simulink model "Inference_only"  (R2022a)
settings: Solver=VariableStepAuto  StartTime=0.0  StopTime=6  RelTol=1e-3
values from neighbouring files (symbols this model uses):
  num_layer = 2    [Inference_only_2x2_input.m]
undefined symbols (not defined in the file or in its folder): xc7k70tfbv676
libraries: hdlBasic x38, vmcUtilities x1
settings Model: Creator=gaozh  LastModifiedBy=gaozh

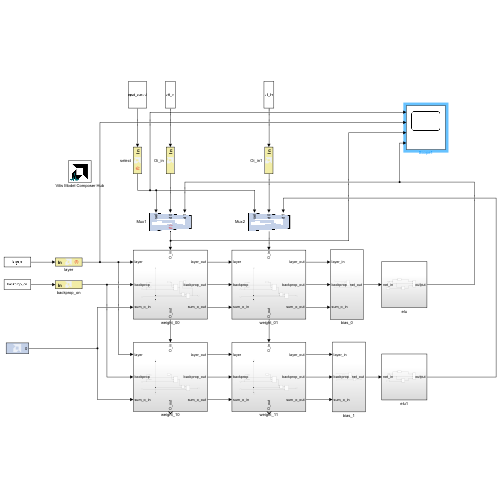
[thumbnail: Simulink's stored preview of the top-level diagram]
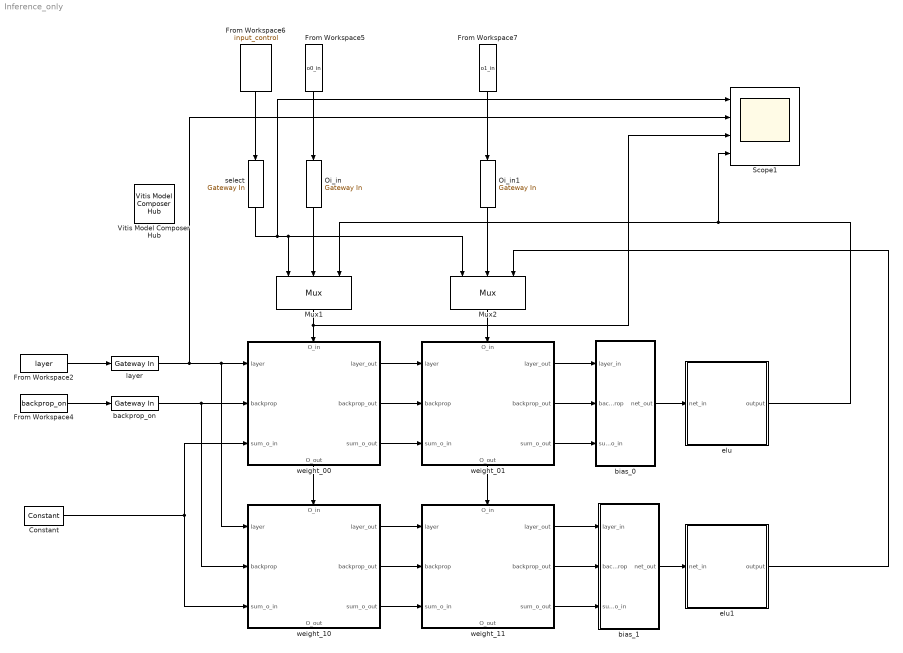
== system Inference_only ==
  Constant : hdlBasic/Constant  const=0  gui_display_data_type=Fixed-point  arith_type=Signed (2's comp)  n_bits=num_bits  bin_pt=frac_bits  preci_type=Single  exp_width=8  frac_width=24  explicit_period=off  period=1  XmcBlockStatus=1  maskContainerNames=tabcontainer1  block_type=constant  block_config=sysgen:Constant_config
  From Workspace2 : FromWorkspace  VariableName=layer
  From Workspace4 : FromWorkspace  VariableName=backprop_on
  From Workspace5 : FromWorkspace  VariableName=o0_in
  From Workspace6 : FromWorkspace  VariableName=input_control  OutputAfterFinalValue=Holding final value
  From Workspace7 : FromWorkspace  VariableName=o1_in
  Mux1 : hdlBasic/Mux  inputs=2  en=off  latency=0  precision=User Defined  arith_type="Signed  (2's comp)"  n_bits=num_bits  bin_pt=frac_bits  quantization=Truncate  overflow=Wrap  XmcBlockStatus=1  maskContainerNames=tabcontainer1  block_type=mux  block_config=sysgen:Mux_config
  Mux2 : hdlBasic/Mux  inputs=2  en=off  latency=0  precision=User Defined  arith_type="Signed  (2's comp)"  n_bits=num_bits  bin_pt=frac_bits  quantization=Truncate  overflow=Wrap  XmcBlockStatus=1  maskContainerNames=tabcontainer1  block_type=mux  block_config=sysgen:Mux_config
  Oi_in : hdlBasic/Gateway In  gui_display_data_type=Fixed-point  arith_type=Signed (2's comp)  n_bits=num_bits  bin_pt=frac_bits  preci_type=Single  exp_width=8  frac_width=24  rows=1  columns=1  quantization="Round  (unbiased: +/- Inf)"  overflow=Saturate  period=1  UseAsADC=off  ADCChannel='1'  interface=None  automatic_assignment=on  address_offset=hex2dec('00')  intf_name=''  intf_description=''  default_value=0  timing_constraint=None  locs_specified=off  LOCs={}  io_standard={}  inherit_from_input=off  hdl_port=on  XmcBlockStatus=1  maskContainerNames=group4  block_type=gatewayin  block_config=sysgen:gateway_in_config  block_width_w=590  block_height_w=620  block_width=640  block_height=850
  Oi_in1 : hdlBasic/Gateway In  gui_display_data_type=Fixed-point  arith_type=Signed (2's comp)  n_bits=num_bits  bin_pt=frac_bits  preci_type=Single  exp_width=8  frac_width=24  rows=1  columns=1  quantization="Round  (unbiased: +/- Inf)"  overflow=Saturate  period=1  UseAsADC=off  ADCChannel='1'  interface=None  automatic_assignment=on  address_offset=hex2dec('00')  intf_name=''  intf_description=''  default_value=0  timing_constraint=None  locs_specified=off  LOCs={}  io_standard={}  inherit_from_input=off  hdl_port=on  XmcBlockStatus=1  maskContainerNames=group4  block_type=gatewayin  block_config=sysgen:gateway_in_config  block_width_w=590  block_height_w=620  block_width=640  block_height=850
  Scope1 : Scope  NumInputPorts=4
  Vitis Model Composer Hub : vmcUtilities/Vitis Model Composer Hub  Tag=genX  CodeGeneration=off  TargetDirectory=./code  ExportType=AI Engines  IpVendor=xilinx.com  IpLibrary=hls  IpVersion=1.0  IpHWLanguage=Verilog  AieCompilerOptions={}  AieSimulatorOptions={}  CreateTestbench=off  TestbenchStackSize=10  RunAieSim=off  AieSimTimeout=50000  RunAieSimProfiling=off  LaunchVitisAnalyzer=off  PlotOutput=off  RunX86Sim=off  X86SimTimeout=10  GenHwImage=off  PlatformType=Not Specified  HwSystemType=Baremetal  HwValidationTarget=hw  ProjDevice=xc7k70tfbv676-1  ProjDevicePart=xc7k70tfbv676-1  SamplePeriod=-1  ClockFrequency=200  DataPathParallelism=1  xilinxfamily=kintex7  part=xc7k70t  speed=-1  package=fbv676  directory=./netlist  testbench=off  incr_netlist=off  synthesis_tool=Vivado  clock_wrapper=Clock Enables  dbl_ovrd=According to Block Masks  dcm_input_clock_period=10  sysclk_period=10  simulink_period=1  eval_field=0  IPInfoJsonString="{\"HDLSubsystem\":{\"SubsystemName\":\"PE_weightstationary\",\"IPName\":\"weight_pe\",\"IPLibrary\":\"VMC\",\"IPVendor\":\"User Company\",\"IPVersion\":\"1.0\"}}"  LogFileName=''  NThreads=4
  backprop_on : hdlBasic/Gateway In  gui_display_data_type=Boolean  arith_type=Boolean  n_bits=num_bits  bin_pt=0  preci_type=Single  exp_width=8  frac_width=24  rows=1  columns=1  quantization="Round  (unbiased: +/- Inf)"  overflow=Saturate  period=1  UseAsADC=off  ADCChannel='1'  interface=None  automatic_assignment=on  address_offset=hex2dec('00')  intf_name=''  intf_description=''  default_value=0  timing_constraint=None  locs_specified=off  LOCs={}  io_standard={}  inherit_from_input=off  hdl_port=on  XmcBlockStatus=1  maskContainerNames=group4  block_type=gatewayin  block_config=sysgen:gateway_in_config  block_width_w=590  block_height_w=620  block_width=640  block_height=850
  bias_0 : Subsystem
  bias_1 : Subsystem
  elu : Subsystem
  elu1 : Subsystem
  layer : hdlBasic/Gateway In  gui_display_data_type=Fixed-point  arith_type=Unsigned  n_bits=ceil(log2(num_layer))  bin_pt=0  preci_type=Single  exp_width=8  frac_width=24  rows=1  columns=1  quantization="Round  (unbiased: +/- Inf)"  overflow=Saturate  period=1  UseAsADC=off  ADCChannel='1'  interface=None  automatic_assignment=on  address_offset=hex2dec('00')  intf_name=''  intf_description=''  default_value=0  timing_constraint=None  locs_specified=off  LOCs={}  io_standard={}  inherit_from_input=off  hdl_port=on  XmcBlockStatus=1  maskContainerNames=group4  block_type=gatewayin  block_config=sysgen:gateway_in_config  block_width_w=590  block_height_w=620  block_width=640  block_height=850
  select : hdlBasic/Gateway In  gui_display_data_type=Fixed-point  arith_type=Unsigned  n_bits=1  bin_pt=0  preci_type=Single  exp_width=8  frac_width=24  rows=1  columns=1  quantization="Round  (unbiased: +/- Inf)"  overflow=Flag as error  period=1  UseAsADC=off  ADCChannel='1'  interface=None  automatic_assignment=on  address_offset=hex2dec('00')  intf_name=''  intf_description=''  default_value=0  timing_constraint=None  locs_specified=off  LOCs={}  io_standard={}  inherit_from_input=off  hdl_port=on  XmcBlockStatus=1  maskContainerNames=group4  block_type=gatewayin  block_config=sysgen:gateway_in_config  block_width_w=590  block_height_w=620  block_width=640  block_height=850
  weight_00 : Subsystem
      settings: PortSchema="{\"entries\":[{\"content\":{\"sides\":[{\"content\":{\"connectorIds\":[\"In1\",\"In2\",\"In3\"]},\"type\":\"ConnectorPlacement.EquallySpacedRectSide\",\"uuid\":\"632a3ded-5b94-406e-b0d8-119737680536\"},{\"content\":{\"connectorIds\":[\"Out1\",\"Out2\",\"Out3\"],\"side\":\"RIGHT\"},\"type\":\"ConnectorPlacement.EquallySpacedRectSide\",\"uuid\":\"c449027c-81bc-4843-8994-fcad26195520\"},{\"content\":{\"connectorIds\":[\"In4\"],\"side\":\"TOP\"},\"type\":\"ConnectorPlacement.EquallySpacedRectSide\",\"uuid\":\"ce3d970d-7335-434e-bfbf-286e0c492397\"},{\"content\":{\"connectorIds\":[\"Out4\"],\"side\":\"BOTTOM\"},\"type\":\"ConnectorPlacement.EquallySpacedRectSide\",\"uuid\":\"bc179919-f31d-4e0a-abc3-bb5ef913c3c8\"}]},\"type\":\"ConnectorPlacement.EquallySpacedConnector\",\"uuid\":\"cad1cfc6-1bed-4a03-a2df-30ebe0a8ed6f\"}],\"packageUris\":[\"http://schema.mathworks.com/mf0/Connector/R2020b\"],\"version\":\"1.0\"}"
  weight_01 : Subsystem
      settings: PortSchema="{\"entries\":[{\"content\":{\"sides\":[{\"content\":{\"connectorIds\":[\"In1\",\"In2\",\"In3\"]},\"type\":\"ConnectorPlacement.EquallySpacedRectSide\",\"uuid\":\"632a3ded-5b94-406e-b0d8-119737680536\"},{\"content\":{\"connectorIds\":[\"Out1\",\"Out2\",\"Out3\"],\"side\":\"RIGHT\"},\"type\":\"ConnectorPlacement.EquallySpacedRectSide\",\"uuid\":\"c449027c-81bc-4843-8994-fcad26195520\"},{\"content\":{\"connectorIds\":[\"In4\"],\"side\":\"TOP\"},\"type\":\"ConnectorPlacement.EquallySpacedRectSide\",\"uuid\":\"ce3d970d-7335-434e-bfbf-286e0c492397\"},{\"content\":{\"connectorIds\":[\"Out4\"],\"side\":\"BOTTOM\"},\"type\":\"ConnectorPlacement.EquallySpacedRectSide\",\"uuid\":\"bc179919-f31d-4e0a-abc3-bb5ef913c3c8\"}]},\"type\":\"ConnectorPlacement.EquallySpacedConnector\",\"uuid\":\"cad1cfc6-1bed-4a03-a2df-30ebe0a8ed6f\"}],\"packageUris\":[\"http://schema.mathworks.com/mf0/Connector/R2020b\"],\"version\":\"1.0\"}"
  weight_10 : Subsystem
      settings: PortSchema="{\"entries\":[{\"content\":{\"sides\":[{\"content\":{\"connectorIds\":[\"In1\",\"In2\",\"In3\"]},\"type\":\"ConnectorPlacement.EquallySpacedRectSide\",\"uuid\":\"632a3ded-5b94-406e-b0d8-119737680536\"},{\"content\":{\"connectorIds\":[\"Out1\",\"Out2\",\"Out3\"],\"side\":\"RIGHT\"},\"type\":\"ConnectorPlacement.EquallySpacedRectSide\",\"uuid\":\"c449027c-81bc-4843-8994-fcad26195520\"},{\"content\":{\"connectorIds\":[\"In4\"],\"side\":\"TOP\"},\"type\":\"ConnectorPlacement.EquallySpacedRectSide\",\"uuid\":\"ce3d970d-7335-434e-bfbf-286e0c492397\"},{\"content\":{\"connectorIds\":[\"Out4\"],\"side\":\"BOTTOM\"},\"type\":\"ConnectorPlacement.EquallySpacedRectSide\",\"uuid\":\"bc179919-f31d-4e0a-abc3-bb5ef913c3c8\"}]},\"type\":\"ConnectorPlacement.EquallySpacedConnector\",\"uuid\":\"cad1cfc6-1bed-4a03-a2df-30ebe0a8ed6f\"}],\"packageUris\":[\"http://schema.mathworks.com/mf0/Connector/R2020b\"],\"version\":\"1.0\"}"
  weight_11 : Subsystem
      settings: PortSchema="{\"entries\":[{\"content\":{\"sides\":[{\"content\":{\"connectorIds\":[\"In1\",\"In2\",\"In3\"]},\"type\":\"ConnectorPlacement.EquallySpacedRectSide\",\"uuid\":\"632a3ded-5b94-406e-b0d8-119737680536\"},{\"content\":{\"connectorIds\":[\"Out1\",\"Out2\",\"Out3\"],\"side\":\"RIGHT\"},\"type\":\"ConnectorPlacement.EquallySpacedRectSide\",\"uuid\":\"c449027c-81bc-4843-8994-fcad26195520\"},{\"content\":{\"connectorIds\":[\"In4\"],\"side\":\"TOP\"},\"type\":\"ConnectorPlacement.EquallySpacedRectSide\",\"uuid\":\"ce3d970d-7335-434e-bfbf-286e0c492397\"},{\"content\":{\"connectorIds\":[\"Out4\"],\"side\":\"BOTTOM\"},\"type\":\"ConnectorPlacement.EquallySpacedRectSide\",\"uuid\":\"bc179919-f31d-4e0a-abc3-bb5ef913c3c8\"}]},\"type\":\"ConnectorPlacement.EquallySpacedConnector\",\"uuid\":\"cad1cfc6-1bed-4a03-a2df-30ebe0a8ed6f\"}],\"packageUris\":[\"http://schema.mathworks.com/mf0/Connector/R2020b\"],\"version\":\"1.0\"}"
  wires:
  From Workspace4/1 -> backprop_on/1
  From Workspace5/1 -> Oi_in/1
  backprop_on/1 -> weight_10/2(backprop), weight_00/2(backprop)
  layer/1 -> weight_10/1(layer), weight_00/1(layer), Scope1/2
  From Workspace7/1 -> Oi_in1/1
  From Workspace2/1 -> layer/1
  Mux2/1 -> weight_01/4(O_in)
  From Workspace6/1 -> select/1
  select/1 -> Scope1/1, Mux2/1, Mux1/1
  Mux1/1 -> weight_00/4(O_in), Scope1/3
  Oi_in/1 -> Mux1/2
  Oi_in1/1 -> Mux2/2
  weight_10/2(backprop_out) -> weight_11/2(backprop)
  weight_00/2(backprop_out) -> weight_01/2(backprop)
  weight_00/3(sum_o_out) -> weight_01/3(sum_o_in)
  weight_00/1(layer_out) -> weight_01/1(layer)
  weight_10/1(layer_out) -> weight_11/1(layer)
  weight_10/3(sum_o_out) -> weight_11/3(sum_o_in)
  weight_01/4(O_out) -> weight_11/4(O_in)
  weight_00/4(O_out) -> weight_10/4(O_in)
  weight_01/1(layer_out) -> bias_0/1(layer_in)
  weight_01/2(backprop_out) -> bias_0/2(backprop)
  weight_01/3(sum_o_out) -> bias_0/3(sum_o_in)
  weight_11/1(layer_out) -> bias_1/1(layer_in)
  weight_11/3(sum_o_out) -> bias_1/3(sum_o_in)
  weight_11/2(backprop_out) -> bias_1/2(backprop)
  bias_1/1(net_out) -> elu1/1(net_in)
  elu/1(output) -> Scope1/4, Mux1/3
  elu1/1(output) -> Mux2/3
  Constant/1 -> weight_10/3(sum_o_in), weight_00/3(sum_o_in)
  bias_0/1(net_out) -> elu/1(net_in)

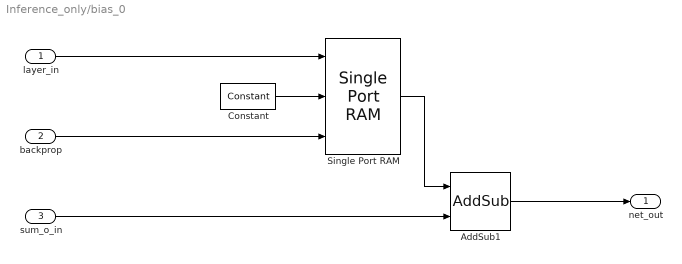
== system Inference_only/bias_0 ==
  layer_in : Inport
  backprop : Inport  Port=2
  sum_o_in : Inport  Port=3
  AddSub1 : hdlBasic/AddSub  mode=Addition  use_carryin=off  use_carryout=off  en=off  latency=0  precision=User Defined  arith_type="Signed  (2's comp)"  n_bits=num_bits  bin_pt=frac_bits  quantization=Truncate  overflow=Saturate  use_behavioral_HDL=off  hw_selection=Fabric  pipelined=off  XmcBlockStatus=1  maskContainerNames=tabcontainer1  block_type=addsub  block_config=sysgen:Addsub_config
  Constant : hdlBasic/Constant  const=0  gui_display_data_type=Fixed-point  arith_type=Signed (2's comp)  n_bits=num_bits  bin_pt=frac_bits  preci_type=Single  exp_width=8  frac_width=24  explicit_period=off  period=1  XmcBlockStatus=1  maskContainerNames=tabcontainer1  block_type=constant  block_config=sysgen:Constant_config
  Single Port RAM : hdlBasic/Single Port RAM  depth=num_layer  initVector=b1  distributed_mem=Block RAM  write_mode=Read After Write  rst=off  init_reg=0  en=off  optimize_latency=off  latency=1  optimize=Area  dbl_ovrd=off  simulation_type=fast_sim  XmcBlockStatus=1  maskContainerNames=tabcontainer1  block_type=spram  block_config=sysgen:SPRAM_config
  net_out : Outport
  wires:
  layer_in/1 -> Single Port RAM/1
  backprop/1 -> Single Port RAM/3
  sum_o_in/1 -> AddSub1/2
  Single Port RAM/1 -> AddSub1/1
  AddSub1/1 -> net_out/1
  Constant/1 -> Single Port RAM/2

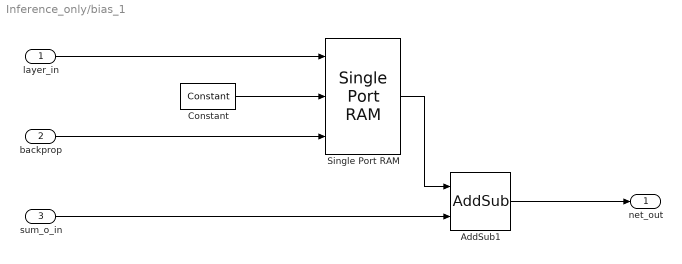
== system Inference_only/bias_1 ==
  layer_in : Inport
  backprop : Inport  Port=2
  sum_o_in : Inport  Port=3
  AddSub1 : hdlBasic/AddSub  mode=Addition  use_carryin=off  use_carryout=off  en=off  latency=0  precision=User Defined  arith_type="Signed  (2's comp)"  n_bits=num_bits  bin_pt=frac_bits  quantization=Truncate  overflow=Saturate  use_behavioral_HDL=off  hw_selection=Fabric  pipelined=off  XmcBlockStatus=1  maskContainerNames=tabcontainer1  block_type=addsub  block_config=sysgen:Addsub_config
  Constant : hdlBasic/Constant  const=0  gui_display_data_type=Fixed-point  arith_type=Signed (2's comp)  n_bits=num_bits  bin_pt=frac_bits  preci_type=Single  exp_width=8  frac_width=24  explicit_period=off  period=1  XmcBlockStatus=1  maskContainerNames=tabcontainer1  block_type=constant  block_config=sysgen:Constant_config
  Single Port RAM : hdlBasic/Single Port RAM  depth=num_layer  initVector=b2  distributed_mem=Block RAM  write_mode=Read After Write  rst=off  init_reg=0  en=off  optimize_latency=off  latency=1  optimize=Area  dbl_ovrd=off  simulation_type=fast_sim  XmcBlockStatus=1  maskContainerNames=tabcontainer1  block_type=spram  block_config=sysgen:SPRAM_config
  net_out : Outport
  wires:
  layer_in/1 -> Single Port RAM/1
  backprop/1 -> Single Port RAM/3
  sum_o_in/1 -> AddSub1/2
  Single Port RAM/1 -> AddSub1/1
  AddSub1/1 -> net_out/1
  Constant/1 -> Single Port RAM/2

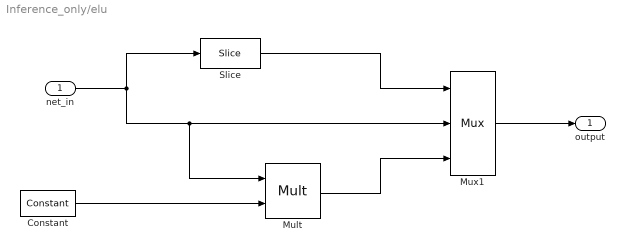
== system Inference_only/elu ==
  net_in : Inport
  Constant : hdlBasic/Constant  const=0.03  gui_display_data_type=Fixed-point  arith_type=Signed (2's comp)  n_bits=num_bits  bin_pt=frac_bits  preci_type=Single  exp_width=8  frac_width=24  explicit_period=off  period=1  XmcBlockStatus=1  maskContainerNames=tabcontainer1  block_type=constant  block_config=sysgen:Constant_config
  Mult : hdlBasic/Mult  precision=User Defined  arith_type="Signed  (2's comp)"  n_bits=num_bits  bin_pt=3  quantization=Truncate  overflow=Wrap  en=off  latency=0  use_behavioral_HDL=off  opt=Speed  use_embedded=on  optimum_pipeline=off  pipeline=on  use_rpm=on  placement_style=Triangular  XmcBlockStatus=1  maskContainerNames=group1  block_type=mult  block_config=sysgen:Mult_config  block_width=598  block_height=876
  Mux1 : hdlBasic/Mux  inputs=2  en=off  latency=1  precision=User Defined  arith_type="Signed  (2's comp)"  n_bits=num_bits  bin_pt=3  quantization=Truncate  overflow=Wrap  XmcBlockStatus=1  maskContainerNames=tabcontainer1  block_type=mux  block_config=sysgen:Mux_config
  Slice : hdlBasic/Slice  nbits=1  boolean_output=on  mode=Upper Bit Location + Width  bit1=0  base1=MSB of Input  bit0=0  base0=LSB of Input  XmcBlockStatus=1  maskContainerNames=group1  block_type=slice  block_config=sysgen:Slice_config
  output : Outport
  wires:
  Mult/1 -> Mux1/3
  Constant/1 -> Mult/2
  Slice/1 -> Mux1/1
  net_in/1 -> Slice/1, Mux1/2, Mult/1
  Mux1/1 -> output/1

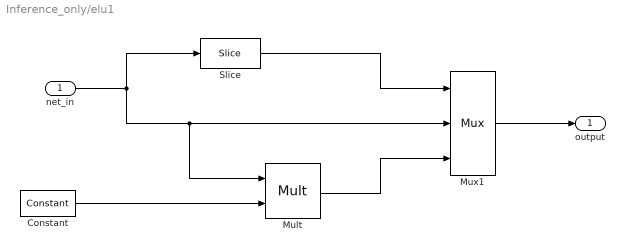
== system Inference_only/elu1 ==
  net_in : Inport
  Constant : hdlBasic/Constant  const=0.03  gui_display_data_type=Fixed-point  arith_type=Signed (2's comp)  n_bits=num_bits  bin_pt=frac_bits  preci_type=Single  exp_width=8  frac_width=24  explicit_period=off  period=1  XmcBlockStatus=1  maskContainerNames=tabcontainer1  block_type=constant  block_config=sysgen:Constant_config
  Mult : hdlBasic/Mult  precision=User Defined  arith_type="Signed  (2's comp)"  n_bits=num_bits  bin_pt=3  quantization=Truncate  overflow=Wrap  en=off  latency=0  use_behavioral_HDL=off  opt=Speed  use_embedded=on  optimum_pipeline=off  pipeline=on  use_rpm=on  placement_style=Triangular  XmcBlockStatus=1  maskContainerNames=group1  block_type=mult  block_config=sysgen:Mult_config  block_width=598  block_height=876
  Mux1 : hdlBasic/Mux  inputs=2  en=off  latency=1  precision=User Defined  arith_type="Signed  (2's comp)"  n_bits=num_bits  bin_pt=3  quantization=Truncate  overflow=Wrap  XmcBlockStatus=1  maskContainerNames=tabcontainer1  block_type=mux  block_config=sysgen:Mux_config
  Slice : hdlBasic/Slice  nbits=1  boolean_output=on  mode=Upper Bit Location + Width  bit1=0  base1=MSB of Input  bit0=0  base0=LSB of Input  XmcBlockStatus=1  maskContainerNames=group1  block_type=slice  block_config=sysgen:Slice_config
  output : Outport
  wires:
  Mult/1 -> Mux1/3
  Constant/1 -> Mult/2
  Slice/1 -> Mux1/1
  net_in/1 -> Slice/1, Mux1/2, Mult/1
  Mux1/1 -> output/1

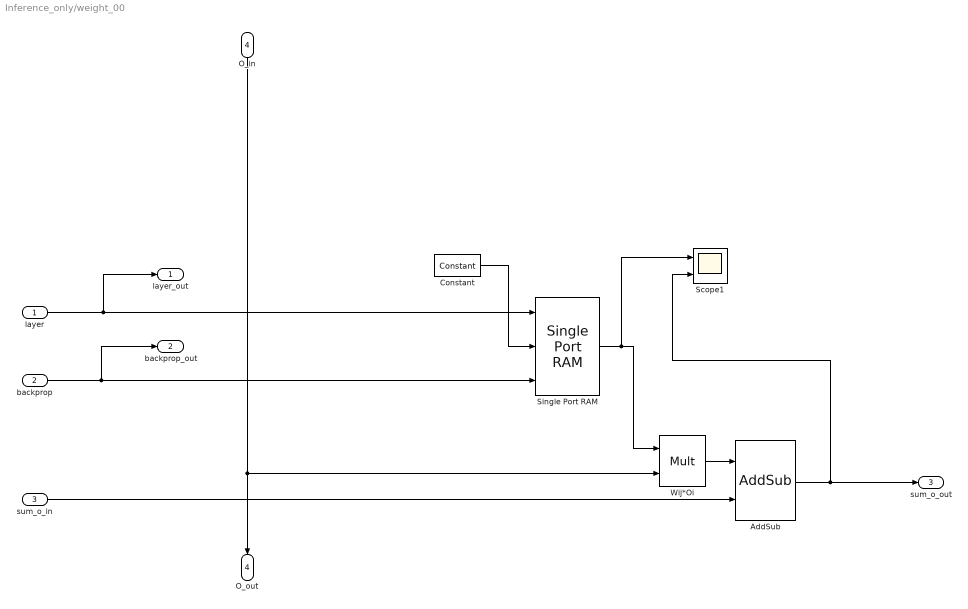
== system Inference_only/weight_00 ==
  layer : Inport
  backprop : Inport  Port=2
  sum_o_in : Inport  Port=3
  O_in : Inport  Port=4
  AddSub : hdlBasic/AddSub  mode=Addition  use_carryin=off  use_carryout=off  en=off  latency=0  precision=User Defined  arith_type="Signed  (2's comp)"  n_bits=num_bits  bin_pt=frac_bits  quantization=Truncate  overflow=Saturate  use_behavioral_HDL=off  hw_selection=Fabric  pipelined=off  XmcBlockStatus=1  maskContainerNames=tabcontainer1  block_type=addsub  block_config=sysgen:Addsub_config
  Constant : hdlBasic/Constant  const=0  gui_display_data_type=Fixed-point  arith_type=Signed (2's comp)  n_bits=num_bits  bin_pt=frac_bits  preci_type=Single  exp_width=8  frac_width=24  explicit_period=off  period=1  XmcBlockStatus=1  maskContainerNames=tabcontainer1  block_type=constant  block_config=sysgen:Constant_config
  Scope1 : Scope  NumInputPorts=2
  Single Port RAM : hdlBasic/Single Port RAM  depth=num_layer  initVector=w00  distributed_mem=Block RAM  write_mode=Read Before Write  rst=off  init_reg=0  en=off  optimize_latency=off  latency=1  optimize=Area  dbl_ovrd=off  simulation_type=fast_sim  XmcBlockStatus=1  maskContainerNames=tabcontainer1  block_type=spram  block_config=sysgen:SPRAM_config
  Wij*Oi : hdlBasic/Mult  precision=User Defined  arith_type="Signed  (2's comp)"  n_bits=num_bits  bin_pt=frac_bits  quantization=Truncate  overflow=Saturate  en=off  latency=0  use_behavioral_HDL=off  opt=Speed  use_embedded=on  optimum_pipeline=off  pipeline=on  use_rpm=on  placement_style=Triangular  XmcBlockStatus=1  maskContainerNames=group1  block_type=mult  block_config=sysgen:Mult_config  block_width=598  block_height=876
  layer_out : Outport
  backprop_out : Outport  Port=2
  sum_o_out : Outport  Port=3
  O_out : Outport  Port=4
  wires:
  O_in/1 -> Wij*Oi/2, O_out/1
  Single Port RAM/1 -> Scope1/1, Wij*Oi/1
  Wij*Oi/1 -> AddSub/1
  sum_o_in/1 -> AddSub/2
  AddSub/1 -> Scope1/2, sum_o_out/1
  backprop/1 -> Single Port RAM/3, backprop_out/1
  layer/1 -> Single Port RAM/1, layer_out/1
  Constant/1 -> Single Port RAM/2

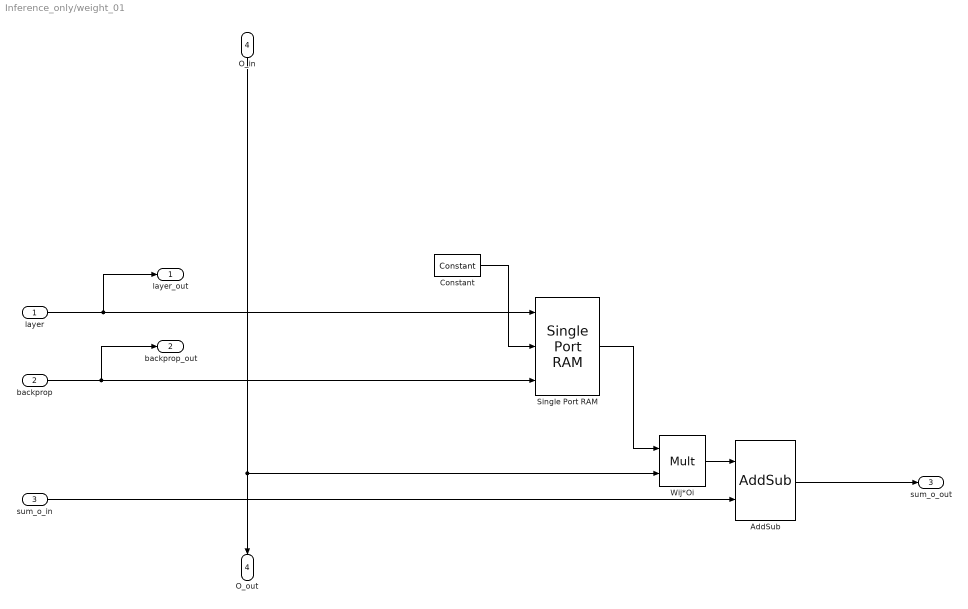
== system Inference_only/weight_01 ==
  layer : Inport
  backprop : Inport  Port=2
  sum_o_in : Inport  Port=3
  O_in : Inport  Port=4
  AddSub : hdlBasic/AddSub  mode=Addition  use_carryin=off  use_carryout=off  en=off  latency=0  precision=User Defined  arith_type="Signed  (2's comp)"  n_bits=num_bits  bin_pt=frac_bits  quantization=Truncate  overflow=Saturate  use_behavioral_HDL=off  hw_selection=Fabric  pipelined=off  XmcBlockStatus=1  maskContainerNames=tabcontainer1  block_type=addsub  block_config=sysgen:Addsub_config
  Constant : hdlBasic/Constant  const=0  gui_display_data_type=Fixed-point  arith_type=Signed (2's comp)  n_bits=num_bits  bin_pt=frac_bits  preci_type=Single  exp_width=8  frac_width=24  explicit_period=off  period=1  XmcBlockStatus=1  maskContainerNames=tabcontainer1  block_type=constant  block_config=sysgen:Constant_config
  Single Port RAM : hdlBasic/Single Port RAM  depth=num_layer  initVector=w01  distributed_mem=Block RAM  write_mode=Read Before Write  rst=off  init_reg=0  en=off  optimize_latency=off  latency=1  optimize=Area  dbl_ovrd=off  simulation_type=fast_sim  XmcBlockStatus=1  maskContainerNames=tabcontainer1  block_type=spram  block_config=sysgen:SPRAM_config
  Wij*Oi : hdlBasic/Mult  precision=User Defined  arith_type="Signed  (2's comp)"  n_bits=num_bits  bin_pt=frac_bits  quantization=Truncate  overflow=Saturate  en=off  latency=0  use_behavioral_HDL=off  opt=Speed  use_embedded=on  optimum_pipeline=off  pipeline=on  use_rpm=on  placement_style=Triangular  XmcBlockStatus=1  maskContainerNames=group1  block_type=mult  block_config=sysgen:Mult_config  block_width=598  block_height=876
  layer_out : Outport
  backprop_out : Outport  Port=2
  sum_o_out : Outport  Port=3
  O_out : Outport  Port=4
  wires:
  O_in/1 -> Wij*Oi/2, O_out/1
  Single Port RAM/1 -> Wij*Oi/1
  Wij*Oi/1 -> AddSub/1
  sum_o_in/1 -> AddSub/2
  AddSub/1 -> sum_o_out/1
  backprop/1 -> Single Port RAM/3, backprop_out/1
  layer/1 -> Single Port RAM/1, layer_out/1
  Constant/1 -> Single Port RAM/2

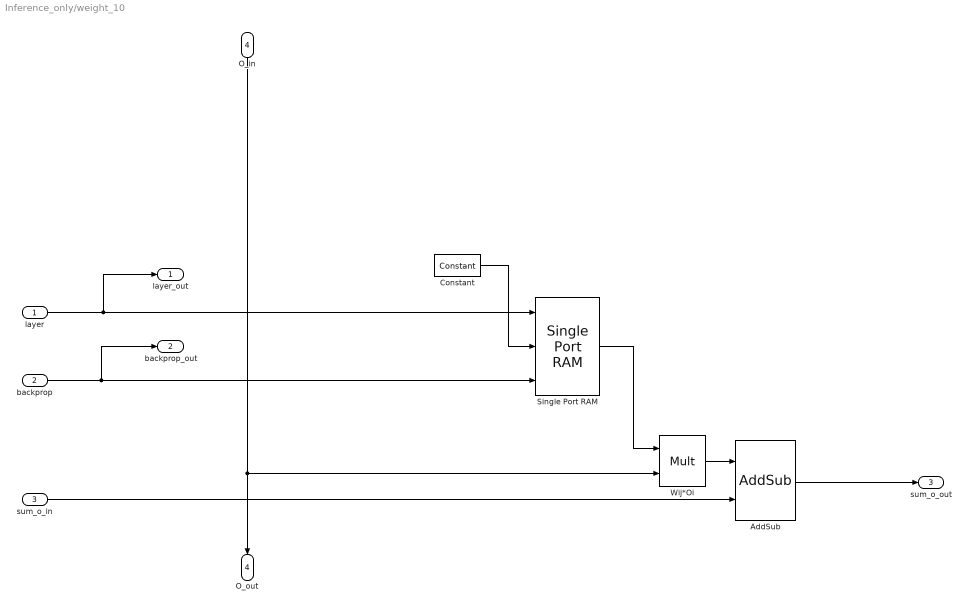
== system Inference_only/weight_10 ==
  layer : Inport
  backprop : Inport  Port=2
  sum_o_in : Inport  Port=3
  O_in : Inport  Port=4
  AddSub : hdlBasic/AddSub  mode=Addition  use_carryin=off  use_carryout=off  en=off  latency=0  precision=User Defined  arith_type="Signed  (2's comp)"  n_bits=num_bits  bin_pt=frac_bits  quantization=Truncate  overflow=Saturate  use_behavioral_HDL=off  hw_selection=Fabric  pipelined=off  XmcBlockStatus=1  maskContainerNames=tabcontainer1  block_type=addsub  block_config=sysgen:Addsub_config
  Constant : hdlBasic/Constant  const=0  gui_display_data_type=Fixed-point  arith_type=Signed (2's comp)  n_bits=num_bits  bin_pt=frac_bits  preci_type=Single  exp_width=8  frac_width=24  explicit_period=off  period=1  XmcBlockStatus=1  maskContainerNames=tabcontainer1  block_type=constant  block_config=sysgen:Constant_config
  Single Port RAM : hdlBasic/Single Port RAM  depth=num_layer  initVector=w10  distributed_mem=Block RAM  write_mode=Read Before Write  rst=off  init_reg=0  en=off  optimize_latency=off  latency=1  optimize=Area  dbl_ovrd=off  simulation_type=fast_sim  XmcBlockStatus=1  maskContainerNames=tabcontainer1  block_type=spram  block_config=sysgen:SPRAM_config
  Wij*Oi : hdlBasic/Mult  precision=User Defined  arith_type="Signed  (2's comp)"  n_bits=num_bits  bin_pt=frac_bits  quantization=Truncate  overflow=Saturate  en=off  latency=0  use_behavioral_HDL=off  opt=Speed  use_embedded=on  optimum_pipeline=off  pipeline=on  use_rpm=on  placement_style=Triangular  XmcBlockStatus=1  maskContainerNames=group1  block_type=mult  block_config=sysgen:Mult_config  block_width=598  block_height=876
  layer_out : Outport
  backprop_out : Outport  Port=2
  sum_o_out : Outport  Port=3
  O_out : Outport  Port=4
  wires:
  O_in/1 -> Wij*Oi/2, O_out/1
  Single Port RAM/1 -> Wij*Oi/1
  Wij*Oi/1 -> AddSub/1
  sum_o_in/1 -> AddSub/2
  AddSub/1 -> sum_o_out/1
  backprop/1 -> Single Port RAM/3, backprop_out/1
  layer/1 -> Single Port RAM/1, layer_out/1
  Constant/1 -> Single Port RAM/2

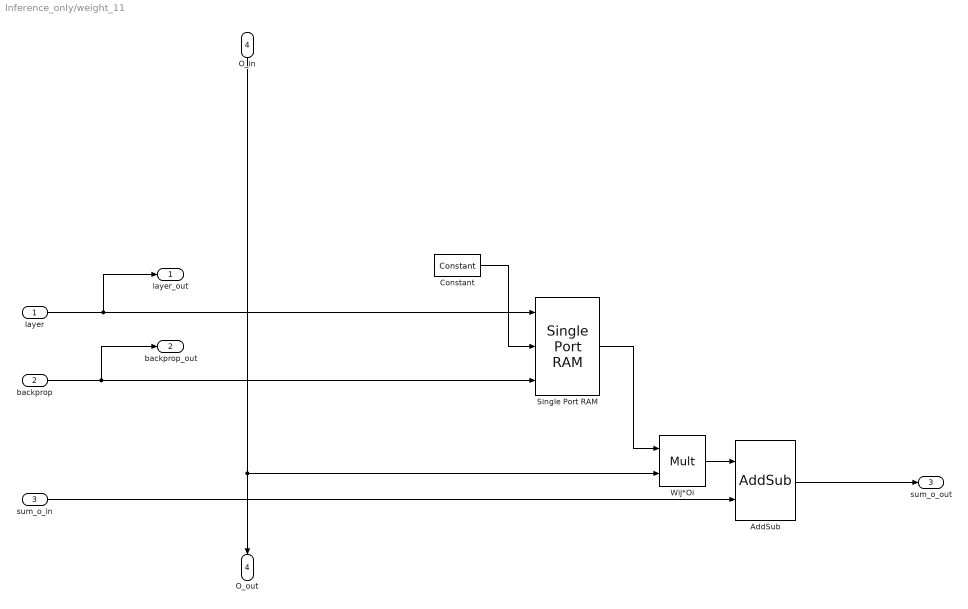
== system Inference_only/weight_11 ==
  layer : Inport
  backprop : Inport  Port=2
  sum_o_in : Inport  Port=3
  O_in : Inport  Port=4
  AddSub : hdlBasic/AddSub  mode=Addition  use_carryin=off  use_carryout=off  en=off  latency=0  precision=User Defined  arith_type="Signed  (2's comp)"  n_bits=num_bits  bin_pt=frac_bits  quantization=Truncate  overflow=Saturate  use_behavioral_HDL=off  hw_selection=Fabric  pipelined=off  XmcBlockStatus=1  maskContainerNames=tabcontainer1  block_type=addsub  block_config=sysgen:Addsub_config
  Constant : hdlBasic/Constant  const=0  gui_display_data_type=Fixed-point  arith_type=Signed (2's comp)  n_bits=num_bits  bin_pt=frac_bits  preci_type=Single  exp_width=8  frac_width=24  explicit_period=off  period=1  XmcBlockStatus=1  maskContainerNames=tabcontainer1  block_type=constant  block_config=sysgen:Constant_config
  Single Port RAM : hdlBasic/Single Port RAM  depth=num_layer  initVector=w11  distributed_mem=Block RAM  write_mode=Read Before Write  rst=off  init_reg=0  en=off  optimize_latency=off  latency=1  optimize=Area  dbl_ovrd=off  simulation_type=fast_sim  XmcBlockStatus=1  maskContainerNames=tabcontainer1  block_type=spram  block_config=sysgen:SPRAM_config
  Wij*Oi : hdlBasic/Mult  precision=User Defined  arith_type="Signed  (2's comp)"  n_bits=num_bits  bin_pt=frac_bits  quantization=Truncate  overflow=Saturate  en=off  latency=0  use_behavioral_HDL=off  opt=Speed  use_embedded=on  optimum_pipeline=off  pipeline=on  use_rpm=on  placement_style=Triangular  XmcBlockStatus=1  maskContainerNames=group1  block_type=mult  block_config=sysgen:Mult_config  block_width=598  block_height=876
  layer_out : Outport
  backprop_out : Outport  Port=2
  sum_o_out : Outport  Port=3
  O_out : Outport  Port=4
  wires:
  O_in/1 -> Wij*Oi/2, O_out/1
  Single Port RAM/1 -> Wij*Oi/1
  Wij*Oi/1 -> AddSub/1
  sum_o_in/1 -> AddSub/2
  AddSub/1 -> sum_o_out/1
  backprop/1 -> Single Port RAM/3, backprop_out/1
  layer/1 -> Single Port RAM/1, layer_out/1
  Constant/1 -> Single Port RAM/2
